simulink model "xhblock1"  (Simulink 2.20)
settings: Solver=ode45  StartTime=0.0  StopTime=10.0  RelTol=1e-3  AbsTol=1e-6
undefined symbols (not defined in the file): offset, ssfunpsd
settings Model: ConsistencyChecking=off  RTWPlaceOutputsASAP=off

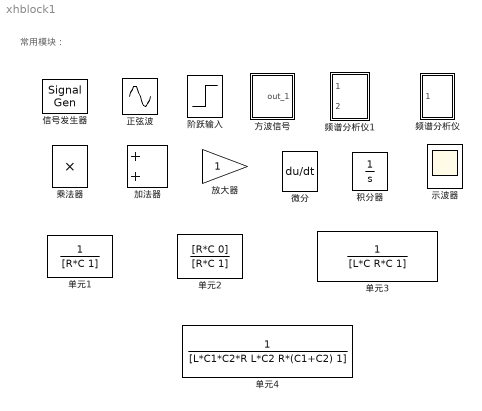
== system xhblock1 ==
  note: 常用模块：
  乘法器 : Product  Inputs=2
  单元1 : TransferFcn  Numerator=[1]  Denominator=[R*C 1]  mask(积分 1],, 2065, 291]){}
      mask help: 积分 1],, 2065, 291]
      mask init:
      | C=@1;R=@2;
      mask Display: plot([0 2 2 2],[2 2 1.5 2.5],[2 6],[2.5 2.5],[2 6],[1.5 1.5],[6 6],[2.5 1.5],[6 11],[2 2],[8 8 6 10],[2 0 0 0],[6 10],[-1 -1],[8 8 7 9],[-1 -3 -3 -3]);
  单元2 : TransferFcn  Numerator=[R*C 0]  Denominator=[R*C 1]  mask(微分 1]3, 1995, 292]){}
      mask help: 微分 1]3, 1995, 292]
      mask init:
      | C=@1;R=@2;
      mask Display: plot([0 2 2 2],[2 2 0 4],[3 3 3 8],[0 4 2 2],[6 6 5.5 6.5],[2 0 0 0],[5.5 5.5],[0 -4],[6.5 6.5],[0 -4],[5.5 6.5 6 6],[-4 -4 -4 -5.5],[5.5 6.5],[-5.5 -5.5]);
  单元3 : TransferFcn  Numerator=[1]  Denominator=[L*C R*C 1]  mask( 单元7*C 1]65,, 295]0 ){}
      mask help: 单元7*C 1]65,, 295]0
      mask init:
      | R=@1;L=@2;C=@3;
      mask Display: plot([3 5 5 5],[2 2 1.5 2.5],[5 9],[2.5 2.5],[5 9],[1.5 1.5],[9 9],[2.5 1.5],[9 11],[2 2],[11:1/7:12],[2 2.5 2.707 2.866 2.866 2.707 2.5 2],[12:1/7:13],[2 2.5 2.707 2.866 2.866 2.707 2.5 2],[13:1/7:14],[2 2.5 2.707 2.866 2.866 2.707 2.5 2],[14:1/7:15],[2 2.5 2.707 2.866 2.866 2.707 2.5 2],[15 21],[2 2],[18 18 16 20],[2 0 0 0],[16 20],[-1 -1],[18 18 17 19],[-1 -3 -3 -3]);
  单元4 : TransferFcn  Numerator=[1]  Denominator=[L*C1*C2*R L*C2 R*(C1+C2) 1]  mask(单元5*C2*R L*C2 R*(C1){}
      mask help: 单元5*C2*R L*C2 R*(C1
      mask init:
      | R=@1;C1=@2;L=@3;C2=@4;
      mask Display: plot([0 2 2 2],[2 2 1.5 2.5],[2 6],[2.5 2.5],[2 6],[1.5 1.5],[6 6],[2.5 1.5],[6 11],[2 2],[8 8 6 10],[2 0 0 0],[6 10],[-1 -1],[8 8 7 9],[-1 -3 -3 -3],[11:1/7:12],[2 2.5 2.707 2.866 2.866 2.707 2.5 2],[12:1/7:13],[2 2.5 2.707 2.866 2.866 2.707 2.5 2],[13:1/7:14],[2 2.5 2.707 2.866 2.866 2.707 2.5 2],[14:1/7:15],[2 2.5 2.707 2.866 2.866 2.707 2.5 2],[15 21],[2 2],[18 18 16 20],[2 0 0 0],[16 20],[-1 -1],[18 18 17 19],[-1 -3 -3 -3]);disp('R     C1     L      C2')
  方波信号 : Subsystem  mask(Pulse Generator){}
      mask help: Pulse Generator.
      mask init:
      | Ts=@1; du=@2; ht=@3; stt=@4; ini=ones(length(ht),1); st1=rem(stt,Ts); st2=rem(stt+du,Ts);if(Ts<=1.2*du),ini=zeros(length(ht),1);end;
      mask Help: Pulse generator which ensures pulse\ntransitions are hit. Provides a vector of pulses when the height is entered as a vector.\nUnmask to see how it works.
      mask Display: plot(0,0,100,100,[90,75,75,60,60,35,35,20,20,10],[20,20,80,80,20,20,80,80,20,20])
  放大器 : Gain  Gain=1
  积分器 : Integrator  ExternalReset=none  InitialConditionSource=internal  InitialCondition=0  LimitOutput=off  UpperSaturationLimit=inf  LowerSaturationLimit=-inf  ShowSaturationPort=off  ShowStatePort=off  AbsoluteTolerance=auto
  加法器 : Sum  Inputs=++
  阶跃输入 : Step  Time=1  Before=0  After=1
  频谱分析仪 : Subsystem  LoadFcn=ssfunpsd([],[],[],'LoadBlock')  StartFcn=ssfunpsd([],[],[],'Start')  mask(频谱分析仪],[],[],'NameChange')),35,35,20,20,10],[){}
      mask help: 频谱分析仪（利用图形窗口显示实时结果）5 2.5],[5 9],[1.5 1.5],[9 9],[2.5 1.5],[9 11],[2 2],[11:1/7:12],[2 2.5 2.707length(ht),1);end;k to see how it works.1/7:12],[2 2.5 2.707 2.866 2.866 2.7
      mask init:
      | npts=@1; fftpts=@2; HowOften=@3; ts=@4(1); if length(@4) > 1, offset = @4(2), else, offset = 0; end
      settings: CopyFcn=ssfunpsd([],[],[],'CopyBlock')  DeleteFcn=ssfunpsd([],[],[],'DeleteBlock')  NameChangeFcn=ssfunpsd([],[],[],'NameChange')
      mask Help:
      | µ±°Ñ¸ÃÄ£¿éÁ¬½Óµ½Ò»¸öÏµÍ³µÄÊä³öÊ±£¬½«ÒÔÍ¼ÐÎ´°¿Úµ"
      | ],[1.5 1.5],[9 9],[2.5 1.5],[9 11],[2 2],[11:1/
      mask Display: plot(0,0,100,100,[14,91,91,14,14],[86,86,40,40,86],[85,82,80,79,75,67,63,60,57,53,41,36,33,27,24],[49,50,53,50,49,51,54,66,54,50,50,52,81,51,49])
  "频谱分析仪1 " : Subsystem  mask(Spectrum analyzer.){}
      mask help:
      | Spectrum analyser using graph window.
      | Hook input 1 to system input.
      | Hook input 2 to system output.
      mask init:
      | npts=@1; fftpts=@2; HowOften=@3; ts=@4(1); if length(@4) > 1, offset = @4(2), else, offset = 0; end
      mask Help: Hook the system's input to the first port of this block and the system's output to second port. Results are displayed as the frequency response of this system. Use signals with high harmonic content for best results.
      mask Display: plot(0,0,100,100,[11,93,93,11,11],[90,90,40,40,90],[90,80,72,64,55,45,41,36,20],[50,50,52,59,67,75,78,80,80])
  示波器 : Scope
      settings: TickLabels=on  TimeRange=1.000000  YMin=-1.000000  YMax=1.000000  SaveToWorkspace=off  SaveName=ScopeData
  微分 : Derivative
  信号发生器 : SignalGenerator  WaveForm=sine  Amplitude=1.000000  Frequency=1.000000  Units=rad/sec
  正弦波 : Sin  Amplitude=1  Frequency=1  Phase=0  SampleTime=-1

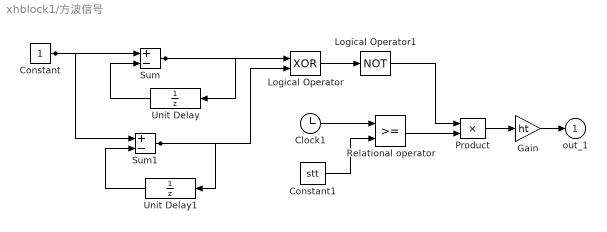
== system xhblock1/方波信号 ==
  Clock1 : Clock
  Constant : Constant  Value=1
  Constant1 : Constant  Value=stt
  Gain : Gain  Gain=ht
  Logical Operator : Logic  Operator=XOR  Inputs=2
  Logical Operator1 : Logic  Operator=NOT  Inputs=1
  Product : Product  Inputs=2
  Relational operator : RelationalOperator  Operator=>=
  Sum : Sum  Inputs=+-
  Sum1 : Sum  Inputs=+-
  Unit Delay : UnitDelay  Orientation=left  X0=0  SampleTime=[Ts,st1]
  Unit Delay1 : UnitDelay  Orientation=left  X0=ini  SampleTime=[Ts,st2]
  out_1 : Outport  Port=1
  wires:
  Logical Operator1/1 -> Product/1
  Logical Operator/1 -> Logical Operator1/1
  Constant1/1 -> Relational operator/2
  Gain/1 -> out_1/1
  Product/1 -> Gain/1
  Relational operator/1 -> Product/2
  Clock1/1 -> Relational operator/1
  Unit Delay/1 -> Sum/2
  Sum/1 -> Unit Delay/1, Logical Operator/1
  Constant/1 -> Sum/1, Sum1/1
  Sum1/1 -> Unit Delay1/1, Logical Operator/2
  Unit Delay1/1 -> Sum1/2

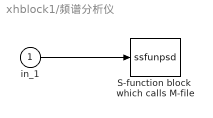
== system xhblock1/频谱分析仪 ==
  in_1 : Inport  Port=1  PortWidth=-1  SampleTime=-1
  S-function block  which calls M-file : S-Function  FunctionName=ssfunpsd  Parameters=fftpts,npts,HowOften,offset,ts,0  PortCounts=[]  SFunctionModules=''
  wires:
  in_1/1 -> S-function block  which calls M-file/1

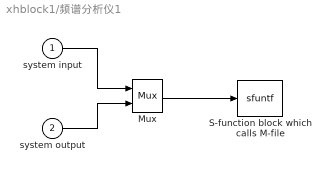
== system xhblock1/频谱分析仪1  ==
  system input : Inport  Port=1  PortWidth=-1  SampleTime=-1
  system output : Inport  Port=2  PortWidth=-1  SampleTime=-1
  Mux : Mux  Inputs=2
  S-function block which calls M-file : S-Function  FunctionName=sfuntf  Parameters=fftpts,npts,HowOften,offset,ts,0  PortCounts=[]  SFunctionModules=''
  wires:
  system output/1 -> Mux/2
  system input/1 -> Mux/1
  Mux/1 -> S-function block which calls M-file/1
